simulink model "P06"  (R2023a)
settings: Solver=VariableStepAuto  StartTime=0.0  StopTime=10.0  RelTol=1e-3
settings Model: Creator=pmt1554  LastModifiedBy=pmt1554

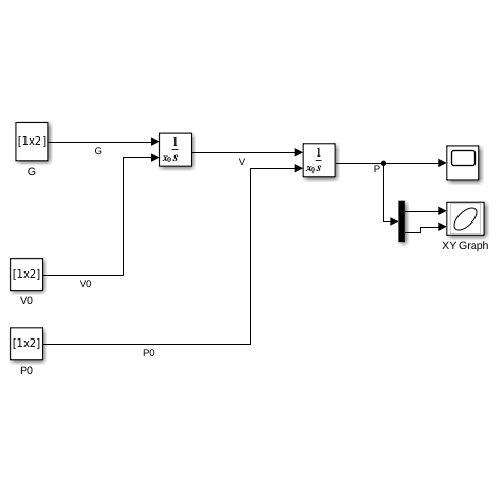
[thumbnail: Simulink's stored preview of the top-level diagram]
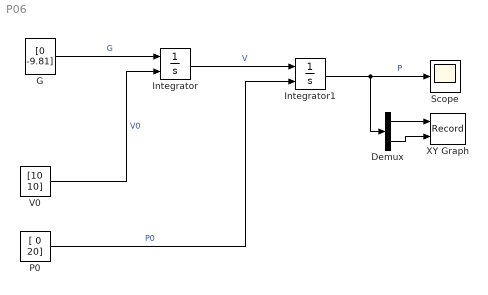
== system P06 ==
  Demux : Demux  Outputs=2
  G : Constant  Value=[0 -9.81]
  Integrator : Integrator  InitialConditionSource=external
  Integrator1 : Integrator  InitialConditionSource=external
  P0 : Constant  Value=[ 0 20]
  Scope : Scope
  V0 : Constant  Value=[10 10]
  XY Graph : Record  FileSettingsInternal="{\"entries\":[{\"content\":{\"excelSettings\":{\"content\":{},\"type\":\"Streamout.ExcelSettings\"}},\"type\":\"Streamout.FileSettingStorage\",\"uuid\":\"a0f425b0-ebbe-4968-ab98-86940a4a1aed\"}],\"packageUris\":[\"http://schema.mathworks.com/mf0/streamout_blocks/R2020a\"],\"version\":\"1.0\"}"  Layout=[1 1]  SignalsInternal="{\"entries\":[{\"content\":{\"signals\":[{\"content\":{\"blockPath\":[\"untitled/XY Graph\"],\"dimensions\":[1],\"domain\":\"untitled/XY Graph\",\"lineColor\":\"#a2142f\",\"plots\":[1],\"port\":1,\"sid\":[\"\"],\"signalID\":27,\"signalName\":\"Demux:1\"},\"type\":\"RecordBlkView.Signal\",\"uuid\":\"071fe151-4e44-4005-a80f-0b80a40e2e0b\"},{\"content\":{\"blockPath\":[\"untitled/XY Graph\"],\"dimensions\":[1],\"domain\":\"untitled/XY Graph\",\"lineColor\":\"#139fff\",\"plots\":[1],\"port\":2,\"sid\":[\"\"],\"signalID\":31,\"signalName\":\"Demux:2\"},\"type\":\"RecordBlkView.Signal\",\"uuid\":\"842e5e6a-f154-4a70-b5f5-b9b69907ef0e\"}]},\"type\":\"RecordBlkView.InputSignals\",\"uuid\":\"36d6462a-bbce-4095-94ea-29b110894e7e\"}],\"packageUris\":[\"http://schema.mathworks.com/mf0/streamout_blocks/R2020a\"],\"version\":\"1.0\"}"  VisualizationBindings="{\"xyplotplugin\":{\"info\":[{\"series\":[{\"bindingParametersList\":[{\"parameter\":\"X-Axis\",\"signalID\":27,\"signalName\":\"Demux:1\"},{\"parameter\":\"Y-Axis\",\"signalID\":31,\"signalName\":\"Demux:2\"}],\"seriesID\":3011}],\"subplotID\":1}]}}"  CompatibilityTag=XY
  wires:
  V0/1 -> Integrator/2  "V0"
  P0/1 -> Integrator1/2  "P0"
  G/1 -> Integrator/1  "G"
  Integrator/1 -> Integrator1/1  "V"
  Integrator1/1 -> Demux/1, Scope/1  "P"
  Demux/1 -> XY Graph/1
  Demux/2 -> XY Graph/2
